simulink model "Sistema_camera"  (R2015a)
settings: Solver=FixedStepDiscrete  StartTime=0.0  StopTime=9  FixedStep=.03  RelTol=1e-3
libraries: dspvision x2, simulink x2
settings Model: Creator=vmaraccini  LastModifiedBy=Administrator

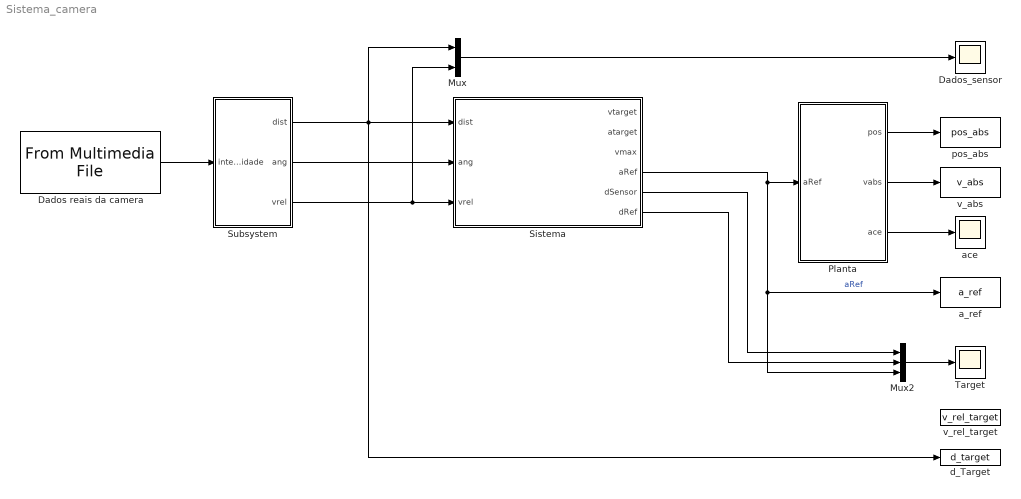
== system Sistema_camera ==
  Dados reais da camera : dspvision/From Multimedia File  inputFilename=\\VBOXSVR\vmaraccini-personal\Documents\MATLAB\TCC\camera-cropped.avi  loop=on  numPlays=1  outputStreams=Video only  videoDataType=double  audioDataType=int16  inheritSampleTime=off  userDefinedSampleTime=.03  noAudioOutput=off  isIntensityVideo=off  fourcc=Intensity  colorVideoFormat=One multidimensional signal  outputEOF=off  dataOrg=Column-major  audioFrameSize=1024  computeAudioFrameSize=off  outSamplingMode=Sample based
  Dados_sensor : Scope
      settings: ShowLegends=on  YMin=-20  YMax=20  SaveName=ScopeData4
  Mux : Mux  Inputs=2
  Mux2 : Mux  Inputs=3
  Planta : Subsystem
  Sistema : Subsystem
  Subsystem : Subsystem
  Target : Scope
      settings: ShowLegends=on  YMin=-4  YMax=6
  a_ref : ToWorkspace  VariableName=a_ref  SaveFormat=Timeseries  SampleTime=-1
  ace : Scope
      settings: SaveName=ScopeData2
  d_Target : ToWorkspace  VariableName=d_target  SaveFormat=Timeseries  SampleTime=-1
  pos_abs : ToWorkspace  VariableName=pos_abs  SaveFormat=Timeseries  SampleTime=-1
  v_abs : ToWorkspace  VariableName=v_abs  SaveFormat=Timeseries  SampleTime=-1
  v_rel_target : ToWorkspace  VariableName=v_rel_target  SaveFormat=Timeseries  SampleTime=-1
  wires:
  Mux2/1 -> Target/1
  Mux/1 -> Dados_sensor/1
  Sistema/5(dSensor) -> Mux2/1
  Sistema/6(dRef) -> Mux2/2
  Sistema/4(aRef) -> Planta/1(aRef), Mux2/3, a_ref/1  "aRef"
  Planta/1(pos) -> pos_abs/1
  Planta/2(vabs) -> v_abs/1
  Planta/3(ace) -> ace/1
  Subsystem/1(dist) -> Mux/1, Sistema/1(dist), d_Target/1
  Dados reais da camera/1 -> Subsystem/1(intensidade)
  Subsystem/3(vrel) -> Sistema/3(vrel), Mux/2
  Subsystem/2(ang) -> Sistema/2(ang)

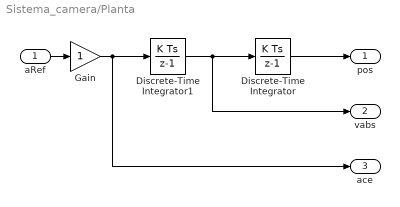
== system Sistema_camera/Planta ==
  aRef : Inport
  Discrete-Time Integrator : DiscreteIntegrator  InitialConditionSetting=State (most efficient)  SampleTime=-1
  Discrete-Time Integrator1 : DiscreteIntegrator  gainval=.2  InitialCondition=10  InitialConditionSetting=State (most efficient)  SampleTime=-1
  Gain : Gain
  pos : Outport
  vabs : Outport  Port=2
  ace : Outport  Port=3
  wires:
  aRef/1 -> Gain/1
  Discrete-Time Integrator/1 -> pos/1
  Discrete-Time Integrator1/1 -> Discrete-Time Integrator/1, vabs/1
  Gain/1 -> Discrete-Time Integrator1/1, ace/1

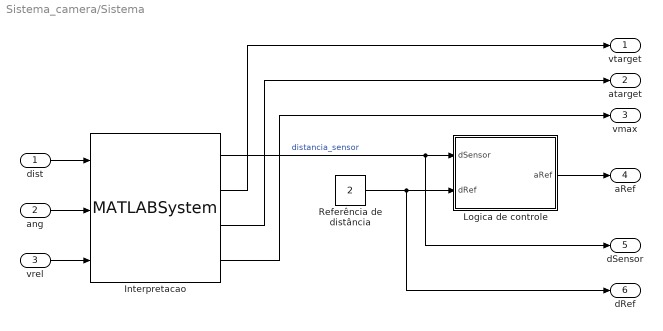
== system Sistema_camera/Sistema ==
  dist : Inport
  ang : Inport  Port=2
  vrel : Inport  Port=3
  Interpretacao : MATLABSystem  System=Interpretacao  SimulateUsing=Interpreted execution
      mask Type: Interpretacao
      mask Display:
      | disp('Interpretacao');
      | port_label('input',1,'dist');
      | port_label('input',2,'ang');
      | port_label('input',3,'vrel');
      | port_label('output',1,'d');
      | port_label('output',2,'v');
      | port_label('output',3,'a');
      | port_label('output',4,'max');
  Logica de controle : Subsystem
  Referência de distância : Constant  Value=2
  vtarget : Outport
  atarget : Outport  Port=2
  vmax : Outport  Port=3
  aRef : Outport  Port=4
  dSensor : Outport  Port=5
  dRef : Outport  Port=6
  wires:
  Interpretacao/2 -> vtarget/1
  Interpretacao/3 -> atarget/1
  dist/1 -> Interpretacao/1
  vrel/1 -> Interpretacao/3
  Interpretacao/4 -> vmax/1
  ang/1 -> Interpretacao/2
  Referência de distância/1 -> Logica de controle/2(dRef), dRef/1
  Interpretacao/1 -> Logica de controle/1(dSensor), dSensor/1  "distancia_sensor"
  Logica de controle/1(aRef) -> aRef/1

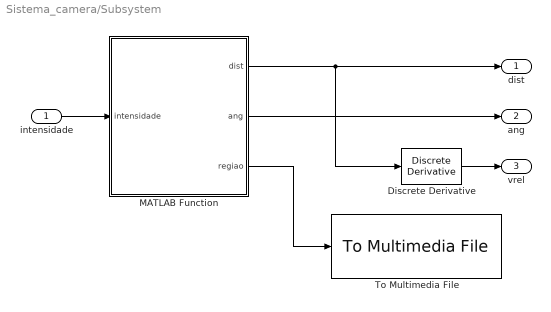
== system Sistema_camera/Subsystem ==
  intensidade : Inport
  Discrete Derivative : simulink/Discrete/Discrete Derivative  gainval=1.0  ICPrevScaledInput=0.0  InputProcessing=Inherited  OutMin=[]  OutMax=[]  OutDataType=fixdt(1, 16)  OutScaling=2^-10  RndMeth=Ceiling  DoSatur=off
  MATLAB Function : MATLAB Function  TreatAsAtomicUnit=on
  To Multimedia File : dspvision/To Multimedia File  outputFilename=output_region.avi  streamSelection=Video only  videoCompressor=None (uncompressed)  audioCompressor=None (uncompressed)  imagePorts=One multidimensional signal  fileType=AVI  audioDatatype=Determine from input data type  fourcc=RGB  videoQuality=75  mj2000CompFactor=10
  dist : Outport
  ang : Outport  Port=2
  vrel : Outport  Port=3
  wires:
  intensidade/1 -> MATLAB Function/1(intensidade)
  MATLAB Function/2(ang) -> ang/1
  Discrete Derivative/1 -> vrel/1
  MATLAB Function/3(regiao) -> To Multimedia File/1
  MATLAB Function/1(dist) -> Discrete Derivative/1, dist/1

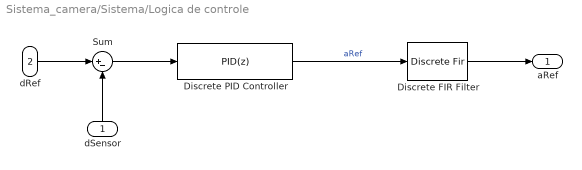
== system Sistema_camera/Sistema/Logica de controle ==
  dSensor : Inport
  dRef : Inport  Port=2
  Discrete FIR Filter : DiscreteFir  Coefficients="[-0,000314745716352413\t-0,000752270719504233\t-0,000521739502826599\t0,00235047230048749\t0,0107169348962010\t0,0271815135910227\t0,0523832412983030\t0,0835978089020548\t0,114679469776097\t0,137791388425939\t0,146351503497156\t0,137791388425939\t0,114679469776097\t0,0835978089020548\t0,0523832412983030\t0,0271815135910227\t0,0107169348962010\t0,00235047230048749\t-0,000521739502826599\t-0,000752270719504233\t-0,000314745716352413]"
  Discrete PID Controller : simulink/Continuous/PID Controller  Controller=PID  TimeDomain=Discrete-time  SampleTime=.03  IntegratorMethod=Forward Euler  FilterMethod=Forward Euler  Form=Parallel  UseFilter=on  ControllerParametersSource=internal  P=-1  I=0  D=-2  N=20  InitialConditionSource=internal  InitialConditionForIntegrator=0  InitialConditionForFilter=0  ExternalReset=none  LimitOutput=off  UpperSaturationLimit=5  LowerSaturationLimit=-2  LinearizeAsGain=off  AntiWindupMode=clamping  Kb=1  TrackingMode=off  Kt=1  PParamMin=[]  PParamMax=[]  IParamMin=[]  IParamMax=[]  DParamMin=[]  DParamMax=[]  NParamMin=[]  NParamMax=[]  KbParamMin=[]  KbParamMax=[]  KtParamMin=[]  KtParamMax=[]  POutMin=[]  POutMax=[]  IOutMin=[]  IOutMax=[]  DOutMin=[]  DOutMax=[]  NOutMin=[]  NOutMax=[]  KbOutMin=[]  KbOutMax=[]  KtOutMin=[]  KtOutMax=[]  IntegratorOutMin=[]  IntegratorOutMax=[]  FilterOutMin=[]  FilterOutMax=[]  SumOutMin=[]  SumOutMax=[]  SumI1OutMin=[]  SumI1OutMax=[]  SumI2OutMin=[]  SumI2OutMax=[]  SumI3OutMin=[]  SumI3OutMax=[]  SumDOutMin=[]  SumDOutMax=[]  SaturationOutMin=[]  SaturationOutMax=[]  IntegratorContinuousStateAttributes=''  IntegratorStateMustResolveToSignalObject=off  IntegratorRTWStateStorageClass=Auto  FilterContinuousStateAttributes=''  FilterStateMustResolveToSignalObject=off  FilterRTWStateStorageClass=Auto  DifferentiatorICPrevScaledInput=0  DifferentiatorOutMin=[]  DifferentiatorOutMax=[]
  Sum : Sum  Inputs=|+-
  aRef : Outport
  wires:
  dSensor/1 -> Sum/2
  Sum/1 -> Discrete PID Controller/1
  dRef/1 -> Sum/1
  Discrete FIR Filter/1 -> aRef/1
  Discrete PID Controller/1 -> Discrete FIR Filter/1  "aRef"

== matlab function Sistema_camera/Subsystem/MATLAB Function ==
  data: intensidade input; dist output; ang output; regiao output
function [dist,ang,regiao] = Adaptador_camera(intensidade)

width = length(intensidade(1,:));
height = length(intensidade(:,1));

hRange = floor(height*.5):ceil(height*.7);
wRange = floor(width*.45):ceil(width*.55);

regiao = intensidade(hRange, wRange);
average = mean(mean(regiao)); %Media da media das colunas

dist = 2*(1 - average);
ang = 0;

end
